simulink model "invertor_simulation"  (R2025a)
settings: Solver=FixedStepAuto  StartTime=0.0  StopTime=150e-3  MaxStep=1e-6  RelTol=1e-3
libraries: spsIGBTDiodeLib x4, spsSeriesRLCBranchLib x2, spsDCVoltageSourceLib x1, spsVoltageMeasurementLib x1, sps_lib x1
settings Model: Creator=natal  LastModifiedBy=natal
settings DataIOCC: ReturnWorkspaceOutputs=off

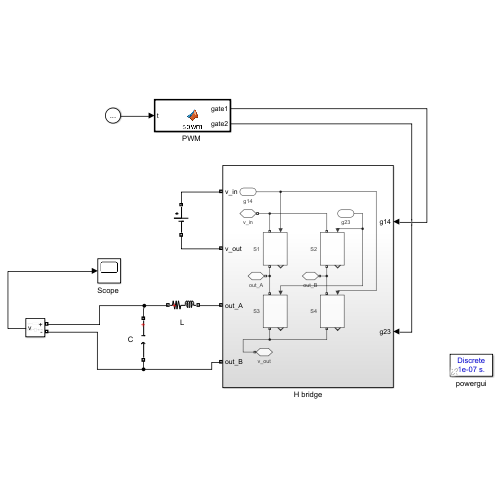
[thumbnail: Simulink's stored preview of the top-level diagram]
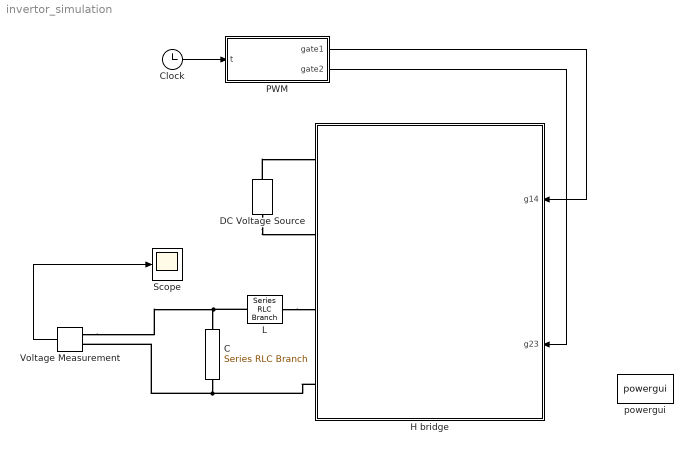
== system invertor_simulation ==
  C : spsSeriesRLCBranchLib/Series RLC Branch  LConnTagsString=__new0  RConnTagsString=__new0  BranchType=C  Resistance=1  Inductance=1e-3  SetiL0=off  InitialCurrent=0  Capacitance=100e-6  Setx0=off  InitialVoltage=0  Measurements=None
  Clock : Clock
  DC Voltage Source : spsDCVoltageSourceLib/DC Voltage Source  Amplitude=400  Measurements=None
  H bridge : Subsystem
  "L " : spsSeriesRLCBranchLib/Series RLC Branch  LConnTagsString=__new0  RConnTagsString=__new0  BranchType=RL  Resistance=1  Inductance=20e-3  SetiL0=off  InitialCurrent=0  Capacitance=1e-6  Setx0=off  InitialVoltage=0  Measurements=None
  "PWM " : MATLAB Function  TreatAsAtomicUnit=on
  "Scope " : Scope
      settings: ActiveDisplayYMinimum=-546.41273839930386  ActiveDisplayYMaximum=636.1728492972004  DataLoggingVariableName=voltage_out
  Voltage Measurement : spsVoltageMeasurementLib/Voltage Measurement  PhasorSimulation=off  OutputType=Complex  PSBequivalent=0
  powergui : sps_lib/powergui  Priority=1  SimulationMode=Discrete  SampleTime=1e-7  frequency=60  Iterations=50  frequencyindice=0  Pbase=100e6  ErrMax=1e-4  UnitsV=kV  UnitsW=MW  buscounter=0  FunctionMessages=off  echomessages=off  EnableUseOfTLC=off  CurrentSourceSwitches=off  DisableSnubberDevices=off  DisableRonSwitches=off  DisableVfSwitches=off  DisplayEquations=off  AutomaticDiscreteSolvers=off  SolverType=Tustin/Backward Euler (TBE)  Interpol=off  ExternalGateDelay=off  methode=off  Ts=100  x0status=blocks  SPID=on  SwTol=0  HookPort=off  NonlinearTolerance=1e-4  nMaxIteration=100  ContinueOnMaxIteration=off  RestoreLinks=warning  ResistiveCurrentMeasurement=off  Frange=[0:2:500]  Ylog=off  Xlog=on  ShowGrid=off  save=off  variable=ZData  structure=0  ZoomFFT=off  StartTime=0.0  cycles=1  DisplayStyle=1  fundamental=60  FreqAxis=off  MaxFrequency=1000  frequencyindicesteady=1  RmsSteady=1  display=off
  wires:
  "PWM "/1(gate1) -> H bridge/1(g14)
  Voltage Measurement/1 -> "Scope "/1
  Clock/1 -> "PWM "/1(t)
  "PWM "/2(gate2) -> H bridge/2(g23)
  connections:
  DC Voltage Source/RConn1 -- H bridge/RConn1
  DC Voltage Source/LConn1 -- H bridge/RConn2
  "L "/RConn1 -- H bridge/RConn3
  "L "/LConn1 -- Voltage Measurement/LConn1 -- C/LConn1
  H bridge/RConn4 -- C/RConn1 -- Voltage Measurement/LConn2

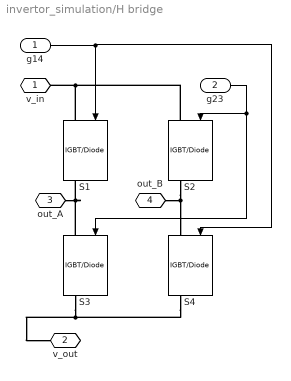
== system invertor_simulation/H bridge ==
  g14 : Inport
  g23 : Inport  Port=2
  S{1..4} (4 alike) : spsIGBTDiodeLib/IGBT//Diode  Ron=1e-3  Rs=1e5  Cs=inf  Measurements=on
  v_in : PMIOPort  Side=Right
  v_out : PMIOPort  Port=2  Side=Right
  out_A : PMIOPort  Port=3  Side=Right
  out_B : PMIOPort  Port=4  Side=Right
  wires:
  g23/1 -> S2/1, S3/1
  g14/1 -> S1/1, S4/1
  connections:
  S3/LConn1 -- out_A/RConn1 -- S1/RConn1
  S2/RConn1 -- out_B/RConn1 -- S4/LConn1
  S1/LConn1 -- S2/LConn1 -- v_in/RConn1
  S3/RConn1 -- S4/RConn1 -- v_out/RConn1

== matlab function invertor_simulation/PWM  ==
  data: t input; gate1 output; gate2 output
function [gate1, gate2] = spwm(t)
    f_ref = 50;             
    f_carrier = 30000;     
    m = 0.85;              
    
    v_ref = m * sin(2 * pi * f_ref * t);
    v_carrier = sawtooth(2 * pi * f_carrier * t, 0.5);

    % Implementacija sa "mrtvom zonom" od 5% amplitude nosioca
    if v_ref > (v_carrier + 0.05)
        gate1 = 1;
        gate2 = 0;
    elseif v_ref < (v_carrier - 0.05)
        gate1 = 0;
        gate2 = 1;
    else
        % DEAD TIME: Ovde su oba tranzistora isključena
        gate1 = 0;
        gate2 = 0;
    end
end
